simulink model "interactive_sample"  (R2014b)
settings: Solver=ode3  StartTime=0.0  StopTime=100  FixedStep=0.1  RelTol=1e-3
settings Model: Creator=Victor  LastModifiedBy=Victor

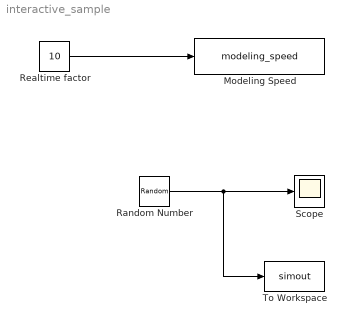
== system interactive_sample ==
  Modeling Speed : S-Function  FunctionName=modeling_speed  EnableBusSupport=off
  Random Number : RandomNumber  Variance=10  SampleTime=0.1
  Realtime factor : Constant  Value=10
  Scope : Scope
      settings: TimeRange=30  YMin=-2.5  YMax=2.5  MaxDataPoints=50000
  To Workspace : ToWorkspace  VariableName=simout  SampleTime=-1
  wires:
  Random Number/1 -> To Workspace/1, Scope/1
  Realtime factor/1 -> Modeling Speed/1
